simulink model "ODE_Hand_Model_v08_IPC_v03"  (Simulink 7.5)
settings: Solver=FixedStepDiscrete  StartTime=0.0  StopTime=inf  FixedStep=0.0315/(4*12)  RelTol=1e-3
values from neighbouring files (symbols this model uses):
  f_step = 0.7    [Set_Parameters.m]
  force_step = 20    [Set_Parameters.m]
  K_Conn = eye(4)*k_conn    [Set_Parameters.m]
  K_D = 30    [Set_Parameters.m]
  K_Or = eye(3)*k_Or    [Set_Parameters.m]
  K_Ot = eye(3)*k_Ot    [Set_Parameters.m]
  K_P = 350    [Set_Parameters.m]
  ksi = 0.9    [Set_Parameters.m]
  Kx = diag([diag(K_Ot)' diag(K_Or)' diag(K_Conn)'])    [Set_Parameters.m]
  l_des = [l1_des; l2_des; l3_des; l4_des]    [Set_Parameters.m]
  Mo = diag([sphere_mass*ones(1,3) (2/5)*sphere_mass*sphere_radius^2*ones(1,3)])    [Set_Parameters.m]
  qd_initial_touch = [0 0.3655   -0.5897   -0.5897     0       -0.3333   +0.5942   +0.5942         0       -0.298   --0.5226   --0.5226           0       -0.3333   +0.5942   +0.5942]    [Set_Parameters.m]
  R_O_Desired = R_O(x_i_v02(qd_initial_touch))    [Set_Parameters.m]
  t_f_start = 2.5    [Set_Parameters.m]
  torque_step = 60    [Set_Parameters.m]
  x_O_desired = (1/4)*sum(x_i_v02(qd_initial_touch))    [Set_Parameters.m]
undefined symbols (not defined in the file or in its folder): sigbuilder_block
libraries: dspmtrx3 x33, simulink x2, dspinverses x1
(part 1 of 6)
settings Model: Creator=konstantinos  LastModifiedBy=konstantinos
settings DataIOCC: SaveOutput=off  SaveTime=off
settings OptimizationCC: SimCompilerOptimization=On
settings SFSimCC: SFSimEnableDebug=off  SFSimOverflowDetection=off

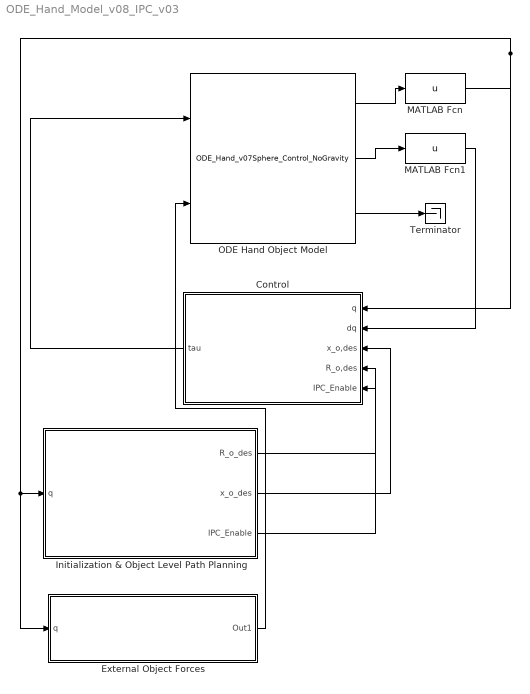
== system ODE_Hand_Model_v08_IPC_v03 ==
  Control : Subsystem
  External Object Forces : Subsystem
  Initialization & Object Level Path Planning : Subsystem
  MATLAB Fcn : MATLABFcn  MATLABFcn=u  Output1D=off
  MATLAB Fcn1 : MATLABFcn  MATLABFcn=u  Output1D=off
  ODE Hand Object Model : S-Function  FunctionName=ODE_Hand_v07Sphere_Control_NoGravity  EnableBusSupport=off
  Terminator : Terminator
  wires:
  Control/1(tau) -> ODE Hand Object Model/1
  Initialization & Object Level Path Planning/2(x_o_des) -> Control/3(x_o,des)
  Initialization & Object Level Path Planning/1(R_o_des) -> Control/4(R_o,des)
  Initialization & Object Level Path Planning/3(IPC_Enable) -> Control/5(IPC_Enable)
  ODE Hand Object Model/3 -> Terminator/1
  External Object Forces/1(Out1) -> ODE Hand Object Model/2
  ODE Hand Object Model/1 -> MATLAB Fcn/1
  MATLAB Fcn/1 -> Initialization & Object Level Path Planning/1(q), External Object Forces/1(q), Control/1(q)
  ODE Hand Object Model/2 -> MATLAB Fcn1/1
  MATLAB Fcn1/1 -> Control/2(dq)

== system ODE_Hand_Model_v08_IPC_v03/Control ==
  q : Inport  OutDataType=fixdt(1, 16)  OutScaling=2^0
  dq : Inport  Port=2  OutDataType=fixdt(1, 16)  OutScaling=2^0
  x_o,des : Inport  Port=3  OutDataType=fixdt(1, 16)  OutScaling=2^0
  R_o,des : Inport  Port=4  OutDataType=fixdt(1, 16)  OutScaling=2^0
  IPC_Enable : Inport  Port=5  OutDataType=fixdt(1, 16)  OutScaling=2^0
  IPC : Subsystem
  Initial_Posture : Subsystem
  Switch : Switch  OutDataType=fixdt(1, 16)  OutScaling=2^0
  tau : Outport  OutDataType=fixdt(1, 16)  OutScaling=2^0
  wires:
  Switch/1 -> tau/1
  x_o,des/1 -> IPC/3(x_o,des)
  R_o,des/1 -> IPC/4(R_o,des)
  IPC/1(tau) -> Switch/1
  IPC_Enable/1 -> Switch/2
  Initial_Posture/1(Out1) -> Switch/3
  q/1 -> IPC/1(q), Initial_Posture/1(q)
  dq/1 -> IPC/2(dq), Initial_Posture/2(dq)

== system ODE_Hand_Model_v08_IPC_v03/External Object Forces ==
  q : Inport  OutDataType=fixdt(1, 16)  OutScaling=2^0
  Apply Force : Subsystem
  Apply Torque : Subsystem
  Display : Display
  Force--Torque : simulink/Signal Routing/Manual Switch  SystemSampleTime=-1  sw=0  action=0  varsize=off
  Gain : Gain  Gain=0  ParameterDataType=fixdt(1, 16)  ParameterScaling=2^0  OutDataType=fixdt(1, 16)  OutScaling=2^0
  Mux1 : Mux
  Mux2 : Mux  Inputs=3
  Mux3 : Mux
  Object Gravity OFF1 : Constant  OutDataType=fixdt(1, 16)  OutScaling=2^0
  Object Gravity ON : Constant  Value=0  OutDataType=fixdt(1, 16)  OutScaling=2^0
  Object_Gravity OFF-ON : simulink/Signal Routing/Manual Switch  SystemSampleTime=-1  sw=1  action=0  varsize=off
  Zero_the Rest : Constant  Value=zeros(1,16-13)  OutDataType=fixdt(1, 16)  OutScaling=2^0
  Out1 : Outport  OutDataType=fixdt(1, 16)  OutScaling=2^0
  wires:
  Object Gravity OFF1/1 -> Object_Gravity OFF-ON/1
  Object Gravity ON/1 -> Object_Gravity OFF-ON/2
  Mux2/1 -> Out1/1, Display/1
  q/1 -> Apply Force/1(In1), Apply Torque/1(In1)
  Zero_the Rest/1 -> Mux2/3
  Object_Gravity OFF-ON/1 -> Mux2/2
  Mux1/1 -> Force--Torque/1
  Mux3/1 -> Force--Torque/2
  Apply Force/1(Out1) -> Mux1/1
  Apply Force/2(Out2) -> Mux1/2
  Apply Force/3(Out3) -> Mux1/3
  Apply Force/4(Out4) -> Mux1/4
  Apply Torque/1(Out1) -> Mux3/1
  Apply Torque/2(Out2) -> Mux3/2
  Apply Torque/3(Out3) -> Mux3/3
  Apply Torque/4(Out4) -> Mux3/4
  Force--Torque/1 -> Gain/1
  Gain/1 -> Mux2/1

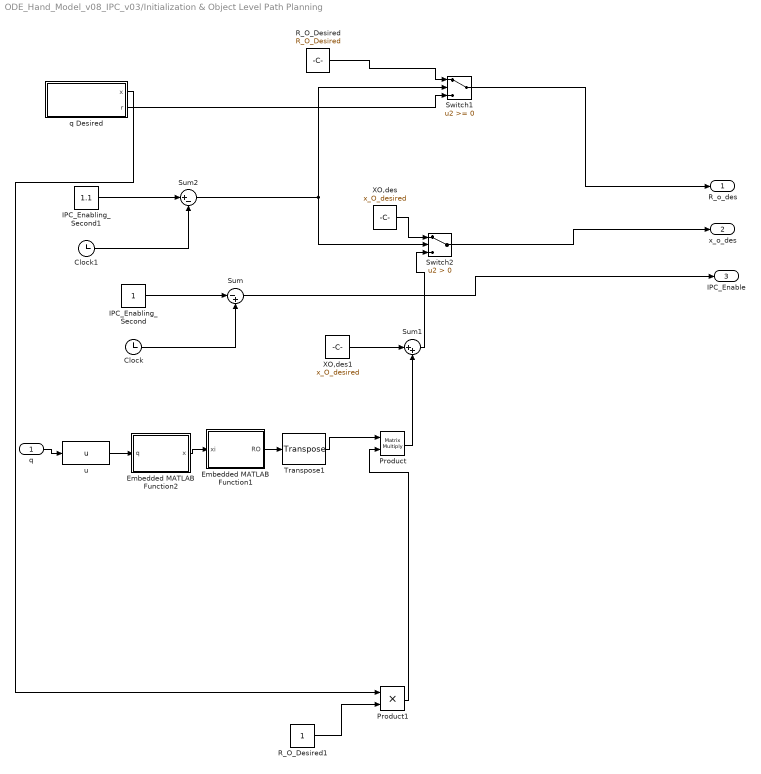
== system ODE_Hand_Model_v08_IPC_v03/Initialization & Object Level Path Planning ==
  q : Inport  OutDataType=fixdt(1, 16)  OutScaling=2^0
  Clock : Clock
      settings: Decimation=10
  Clock1 : Clock
      settings: Decimation=10
  Embedded MATLAB Function1 : Stateflow chart  TreatAsAtomicUnit=on
  Embedded MATLAB Function2 : Stateflow chart  TreatAsAtomicUnit=on
  IPC_Enabling_Second : Constant  OutDataType=fixdt(1, 16)  OutScaling=2^0
  IPC_Enabling_Second1 : Constant  Value=1.1  OutDataType=fixdt(1, 16)  OutScaling=2^0
  Product : Product  Multiplication=Matrix(*)  OutDataType=fixdt(1, 16)  OutScaling=2^0  RndMeth=Zero
  Product1 : Product  OutDataType=fixdt(1, 16)  OutScaling=2^0  RndMeth=Zero
  R_O_Desired : Constant  Value=R_O_Desired  OutDataType=fixdt(1, 16)  OutScaling=2^0
  R_O_Desired1 : Constant  OutDataType=fixdt(1, 16)  OutScaling=2^0
  Sum : Sum  Inputs=|-+  OutDataType=fixdt(1, 16)  OutScaling=2^0
  Sum1 : Sum  Inputs=|++  OutDataType=fixdt(1, 16)  OutScaling=2^0
  Sum2 : Sum  Inputs=|+-  OutDataType=fixdt(1, 16)  OutScaling=2^0
  Switch1 : Switch  OutDataType=fixdt(1, 16)  OutScaling=2^0
  Switch2 : Switch  Criteria=u2 > Threshold  OutDataType=fixdt(1, 16)  OutScaling=2^0
  Transpose1 : dspmtrx3/Transpose  SystemSampleTime=-1  Hermitian=off  overflowFlag=off
  XO,des : Constant  Value=x_O_desired  OutDataType=fixdt(1, 16)  OutScaling=2^0
  XO,des1 : Constant  Value=x_O_desired  OutDataType=fixdt(1, 16)  OutScaling=2^0
  q Desired : Subsystem
  u : MATLABFcn  MATLABFcn=u  Output1D=off
  R_o_des : Outport  OutDataType=fixdt(1, 16)  OutScaling=2^0
  x_o_des : Outport  Port=2  OutDataType=fixdt(1, 16)  OutScaling=2^0
  IPC_Enable : Outport  Port=3  OutDataType=fixdt(1, 16)  OutScaling=2^0
  wires:
  R_O_Desired/1 -> Switch1/1
  Switch2/1 -> x_o_des/1
  q/1 -> u/1
  Embedded MATLAB Function1/1(RO) -> Transpose1/1
  Sum1/1 -> Switch2/3
  XO,des/1 -> Switch2/1
  Product1/1 -> Product/2
  R_O_Desired1/1 -> Product1/2
  u/1 -> Embedded MATLAB Function2/1(q)
  Embedded MATLAB Function2/1(x) -> Embedded MATLAB Function1/1(xi)
  Clock/1 -> Sum/2
  IPC_Enabling_Second/1 -> Sum/1
  Sum/1 -> IPC_Enable/1
  XO,des1/1 -> Sum1/1
  Switch1/1 -> R_o_des/1
  Product/1 -> Sum1/2
  Clock1/1 -> Sum2/2
  IPC_Enabling_Second1/1 -> Sum2/1
  Sum2/1 -> Switch1/2, Switch2/2
  q Desired/1(x) -> Product1/1
  q Desired/2(r) -> Switch1/3
  Transpose1/1 -> Product/1

== system ODE_Hand_Model_v08_IPC_v03/Control/IPC ==
  q : Inport  OutDataType=fixdt(1, 16)  OutScaling=2^0
  dq : Inport  Port=2  OutDataType=fixdt(1, 16)  OutScaling=2^0
  x_o,des : Inport  Port=3  OutDataType=fixdt(1, 16)  OutScaling=2^0
  R_o,des : Inport  Port=4  OutDataType=fixdt(1, 16)  OutScaling=2^0
  Embedded MATLAB Function : Stateflow chart  TreatAsAtomicUnit=on
  Finger Redundancy Controller : Subsystem
  Gain : Gain  Gain=0  ParameterDataType=fixdt(1, 16)  ParameterScaling=2^0  OutDataType=fixdt(1, 16)  OutScaling=2^0
  J : Subsystem
  Object Level Damping(theta) : Subsystem
  "Object Level Stiffnes " : Subsystem
  Sum : Sum  Inputs=|---+  OutDataType=fixdt(1, 16)  OutScaling=2^0
  tau : Outport  OutDataType=fixdt(1, 16)  OutScaling=2^0
  wires:
  q/1 -> Object Level Damping(theta)/1(q), J/1(q), "Object Level Stiffnes "/1(q), Finger Redundancy Controller/1(q), Embedded MATLAB Function/1(theta_in)
  Sum/1 -> tau/1
  dq/1 -> Object Level Damping(theta)/3(dq), Finger Redundancy Controller/2(dq)
  "Object Level Stiffnes "/1(Out1) -> Sum/2
  Object Level Damping(theta)/1(Out1) -> Sum/3
  J/1(J_Ot) -> "Object Level Stiffnes "/2(J_Ot)
  J/2(J_Or) -> "Object Level Stiffnes "/3(J_Or)
  J/4(J_tot) -> Object Level Damping(theta)/2(J_tot)
  Finger Redundancy Controller/1(tau) -> Sum/1
  x_o,des/1 -> J/2(x_o,des), "Object Level Stiffnes "/5(x_o,des)
  J/3(JConn) -> "Object Level Stiffnes "/4(JConn)
  R_o,des/1 -> "Object Level Stiffnes "/6(R_o,des)
  Embedded MATLAB Function/1(gravity_dynamic_term) -> Gain/1
  Gain/1 -> Sum/4

== system ODE_Hand_Model_v08_IPC_v03/Control/Initial_Posture ==
  q : Inport  OutDataType=fixdt(1, 16)  OutScaling=2^0
  dq : Inport  Port=2  OutDataType=fixdt(1, 16)  OutScaling=2^0
  Gain : Gain  Gain=K_P  ParameterDataType=fixdt(1, 16)  ParameterScaling=2^0  OutDataType=fixdt(1, 16)  OutScaling=2^0
  Gain1 : Gain  Gain=K_D  ParameterDataType=fixdt(1, 16)  ParameterScaling=2^0  OutDataType=fixdt(1, 16)  OutScaling=2^0
  Ramp_Singals_qd : Subsystem
  Sum : Sum  Inputs=|--  OutDataType=fixdt(1, 16)  OutScaling=2^0
  Sum1 : Sum  Inputs=|-+  OutDataType=fixdt(1, 16)  OutScaling=2^0
  Out1 : Outport  OutDataType=fixdt(1, 16)  OutScaling=2^0
  wires:
  q/1 -> Sum1/2
  Sum/1 -> Out1/1
  Sum1/1 -> Gain/1
  dq/1 -> Gain1/1
  Gain1/1 -> Sum/1
  Gain/1 -> Sum/2
  Ramp_Singals_qd/1(Out1) -> Sum1/1

== system ODE_Hand_Model_v08_IPC_v03/External Object Forces/Apply Force ==
  In1 : Inport  OutDataType=fixdt(1, 16)  OutScaling=2^0
  Constant : Constant  Value=zeros(1,3)  VectorParams1D=off  OutDataType=fixdt(1, 16)  OutScaling=2^0
  Constant2 : Constant  Value=zeros(1,3)  VectorParams1D=off  OutDataType=fixdt(1, 16)  OutScaling=2^0
  Embedded MATLAB Function : Stateflow chart  TreatAsAtomicUnit=on
  Embedded MATLAB Function1 : Stateflow chart  TreatAsAtomicUnit=on
  Embedded MATLAB Function2 : Stateflow chart  TreatAsAtomicUnit=on
  F_x F_y F_z1 : Subsystem
  Transpose : dspmtrx3/Transpose  SystemSampleTime=-1  Hermitian=off  overflowFlag=off
  Out1 : Outport  OutDataType=fixdt(1, 16)  OutScaling=2^0
  Out2 : Outport  Port=2  OutDataType=fixdt(1, 16)  OutScaling=2^0
  Out3 : Outport  Port=3  OutDataType=fixdt(1, 16)  OutScaling=2^0
  Out4 : Outport  Port=4  OutDataType=fixdt(1, 16)  OutScaling=2^0
  wires:
  F_x F_y F_z1/1(Out1) -> Out2/1
  Embedded MATLAB Function/1(y) -> Out1/1
  Embedded MATLAB Function1/1(RO) -> Transpose/1
  Transpose/1 -> F_x F_y F_z1/1(xi)
  In1/1 -> Embedded MATLAB Function2/1(q)
  Constant/1 -> Out3/1
  Constant2/1 -> Out4/1
  Embedded MATLAB Function2/1(x) -> Embedded MATLAB Function1/1(xi), Embedded MATLAB Function/1(u)

== system ODE_Hand_Model_v08_IPC_v03/External Object Forces/Apply Torque ==
  In1 : Inport  OutDataType=fixdt(1, 16)  OutScaling=2^0
  Subsystem : Subsystem
  Subsystem2 : Subsystem
  Out1 : Outport  OutDataType=fixdt(1, 16)  OutScaling=2^0
  Out2 : Outport  Port=2  OutDataType=fixdt(1, 16)  OutScaling=2^0
  Out3 : Outport  Port=3  OutDataType=fixdt(1, 16)  OutScaling=2^0
  Out4 : Outport  Port=4  OutDataType=fixdt(1, 16)  OutScaling=2^0
  wires:
  Subsystem/1(Out1) -> Out1/1
  Subsystem/2(Out2) -> Out2/1
  Subsystem2/1(Out1) -> Out3/1
  Subsystem2/2(Out2) -> Out4/1
  In1/1 -> Subsystem/1(In1), Subsystem2/1(In1)

== system ODE_Hand_Model_v08_IPC_v03/Initialization & Object Level Path Planning/q Desired ==
  Discrete State-Space : DiscreteStateSpace  A=eye(3)  B=eye(3)  C=eye(3)  D=zeros(3)  X0=zeros(1,3)  SampleTime=0.0315/(4*12)
  Discrete State-Space1 : DiscreteStateSpace  A=eye(3)  B=eye(3)  C=eye(3)  D=zeros(3)  X0=zeros(1,3)  SampleTime=0.0315/(4*12)
  Embedded MATLAB Function : Stateflow chart  TreatAsAtomicUnit=on
  Level-2 M-file S-Function : M-S-Function  FunctionName=sfun_keyboard_input_v1_2
  MATLAB Fcn : MATLABFcn  MATLABFcn=R_O_Desired*rotx(u(1))*roty(u(2))*rotz(u(3))  Output1D=off
  MATLAB Fcn1 : MATLABFcn  MATLABFcn=u
  Product : Product  OutDataType=fixdt(1, 16)  OutScaling=2^0  RndMeth=Zero
  Transpose : dspmtrx3/Transpose  SystemSampleTime=-1  Hermitian=off  overflowFlag=off
  Transpose1 : dspmtrx3/Transpose  SystemSampleTime=-1  Hermitian=off  overflowFlag=off
  x : Outport  OutDataType=fixdt(1, 16)  OutScaling=2^0
  r : Outport  Port=2  OutDataType=fixdt(1, 16)  OutScaling=2^0
  wires:
  Level-2 M-file S-Function/2 -> Product/2
  Level-2 M-file S-Function/1 -> Product/1
  Product/1 -> Embedded MATLAB Function/1(key)
  Discrete State-Space1/1 -> MATLAB Fcn/1
  MATLAB Fcn/1 -> r/1
  MATLAB Fcn1/1 -> x/1
  Embedded MATLAB Function/1(x_f) -> Transpose/1
  Transpose/1 -> Discrete State-Space/1
  Embedded MATLAB Function/2(r_f) -> Transpose1/1
  Discrete State-Space/1 -> MATLAB Fcn1/1
  Transpose1/1 -> Discrete State-Space1/1

== system ODE_Hand_Model_v08_IPC_v03/Control/IPC/Finger Redundancy Controller ==
  q : Inport  OutDataType=fixdt(1, 16)  OutScaling=2^0
  dq : Inport  Port=2  OutDataType=fixdt(1, 16)  OutScaling=2^0
  Embedded MATLAB Function : Stateflow chart  TreatAsAtomicUnit=on
  tau : Outport  OutDataType=fixdt(1, 16)  OutScaling=2^0
  wires:
  dq/1 -> Embedded MATLAB Function/2(dq_in)
  q/1 -> Embedded MATLAB Function/1(q_in)
  Embedded MATLAB Function/1(tau_N) -> tau/1

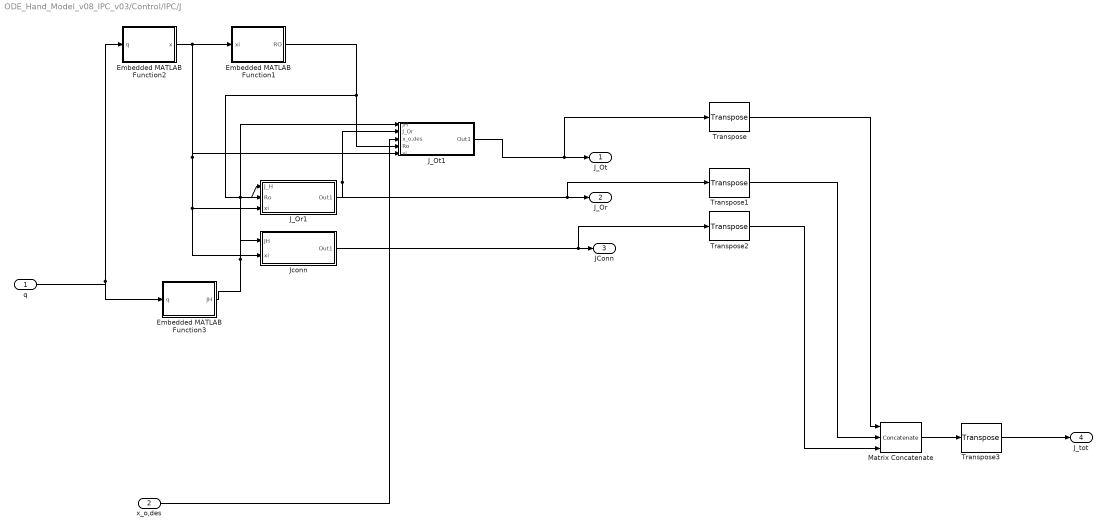
== system ODE_Hand_Model_v08_IPC_v03/Control/IPC/J ==
  q : Inport  OutDataType=fixdt(1, 16)  OutScaling=2^0
  x_o,des : Inport  Port=2  OutDataType=fixdt(1, 16)  OutScaling=2^0
  Embedded MATLAB Function1 : Stateflow chart  TreatAsAtomicUnit=on
  Embedded MATLAB Function2 : Stateflow chart  TreatAsAtomicUnit=on
  Embedded MATLAB Function3 : Stateflow chart  TreatAsAtomicUnit=on
  J_Or1 : Subsystem
  J_Ot1 : Subsystem
  Jconn : Subsystem
  Matrix Concatenate : Concatenate  NumInputs=3  Mode=Multidimensional array  ConcatenateDimension=2
  Transpose{,1..3} (4 alike) : dspmtrx3/Transpose  SystemSampleTime=-1  Hermitian=off  overflowFlag=off
  J_Ot : Outport  OutDataType=fixdt(1, 16)  OutScaling=2^0
  J_Or : Outport  Port=2  OutDataType=fixdt(1, 16)  OutScaling=2^0
  JConn : Outport  Port=3  OutDataType=fixdt(1, 16)  OutScaling=2^0
  J_tot : Outport  Port=4  OutDataType=fixdt(1, 16)  OutScaling=2^0
  wires:
  Embedded MATLAB Function3/1(JH) -> Jconn/1(JH), J_Or1/1(J_H), J_Ot1/1(JH)
  J_Or1/1(Out1) -> J_Ot1/2(J_Or), J_Or/1, Transpose1/1
  q/1 -> Embedded MATLAB Function2/1(q), Embedded MATLAB Function3/1(q)
  J_Ot1/1(Out1) -> J_Ot/1, Transpose/1
  Jconn/1(Out1) -> JConn/1, Transpose2/1
  Transpose2/1 -> Matrix Concatenate/3
  Transpose1/1 -> Matrix Concatenate/2
  Transpose/1 -> Matrix Concatenate/1
  Matrix Concatenate/1 -> Transpose3/1
  Transpose3/1 -> J_tot/1
  x_o,des/1 -> J_Ot1/3(x_o,des)
  Embedded MATLAB Function1/1(RO) -> J_Ot1/4(Ro), J_Or1/2(Ro)
  Embedded MATLAB Function2/1(x) -> J_Ot1/5(xi), J_Or1/3(xi), Jconn/2(xi), Embedded MATLAB Function1/1(xi)

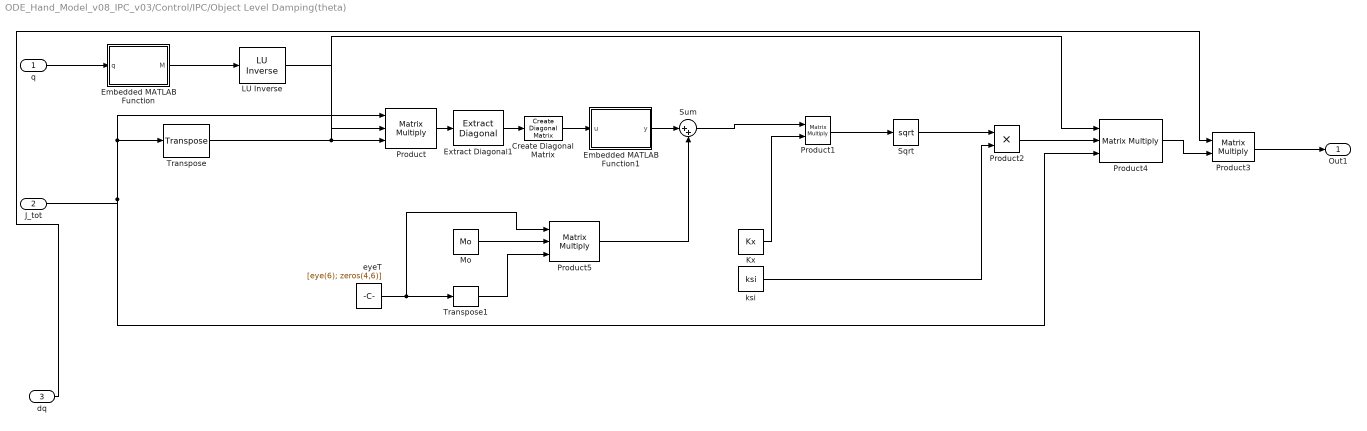
== system ODE_Hand_Model_v08_IPC_v03/Control/IPC/Object Level Damping(theta) ==
  q : Inport  OutDataType=fixdt(1, 16)  OutScaling=2^0
  J_tot : Inport  Port=2  OutDataType=fixdt(1, 16)  OutScaling=2^0
  dq : Inport  Port=3  OutDataType=fixdt(1, 16)  OutScaling=2^0
  " LU Inverse" : dspinverses/ LU Inverse  SystemSampleTime=-1
  Create Diagonal Matrix : dspmtrx3/Create Diagonal Matrix
  Embedded MATLAB Function : Stateflow chart  TreatAsAtomicUnit=on
  Embedded MATLAB Function1 : Stateflow chart  TreatAsAtomicUnit=on
  Extract Diagonal1 : dspmtrx3/Extract Diagonal
  Kx : Constant  Value=Kx  OutDataType=fixdt(1, 16)  OutScaling=2^0
  Mo : Constant  Value=Mo  OutDataType=fixdt(1, 16)  OutScaling=2^0
  Product : Product  Inputs=3  Multiplication=Matrix(*)  OutDataType=fixdt(1, 16)  OutScaling=2^0  RndMeth=Zero
  Product1 : Product  Multiplication=Matrix(*)  OutDataType=fixdt(1, 16)  OutScaling=2^0  RndMeth=Zero
  Product2 : Product  OutDataType=fixdt(1, 16)  OutScaling=2^0  RndMeth=Zero
  Product3 : Product  Multiplication=Matrix(*)  OutDataType=fixdt(1, 16)  OutScaling=2^0  RndMeth=Zero
  Product4 : Product  Inputs=3  Multiplication=Matrix(*)  OutDataType=fixdt(1, 16)  OutScaling=2^0  RndMeth=Zero
  Product5 : Product  Inputs=3  Multiplication=Matrix(*)  OutDataType=fixdt(1, 16)  OutScaling=2^0  RndMeth=Zero
  Sqrt : Sqrt  OutputSignalType=real  SaturateOnIntegerOverflow=on
  Sum : Sum  Inputs=|++  OutDataType=fixdt(1, 16)  OutScaling=2^0
  Transpose : dspmtrx3/Transpose  SystemSampleTime=-1  Hermitian=off  overflowFlag=off
  Transpose1 : dspmtrx3/Transpose  SystemSampleTime=-1  Hermitian=off  overflowFlag=off
  eyeT : Constant  Value=[eye(6); zeros(4,6)]  OutDataType=fixdt(1, 16)  OutScaling=2^0
  ksi : Constant  Value=ksi  OutDataType=fixdt(1, 16)  OutScaling=2^0
  Out1 : Outport  OutDataType=fixdt(1, 16)  OutScaling=2^0
  wires:
  q/1 -> Embedded MATLAB Function/1(q)
  J_tot/1 -> Transpose/1, Product/1, Product4/3
  Transpose/1 -> Product/3, Product4/1
  Embedded MATLAB Function/1(M) -> " LU Inverse"/1
  " LU Inverse"/1 -> Product/2
  Sqrt/1 -> Product2/1
  ksi/1 -> Product2/2
  Product2/1 -> Product4/2
  Product3/1 -> Out1/1
  Kx/1 -> Product1/2
  Product1/1 -> Sqrt/1
  eyeT/1 -> Transpose1/1, Product5/1
  Sum/1 -> Product1/1
  Mo/1 -> Product5/2
  Transpose1/1 -> Product5/3
  Product5/1 -> Sum/2
  Product/1 -> Extract Diagonal1/1
  Extract Diagonal1/1 -> Create Diagonal Matrix/1
  Create Diagonal Matrix/1 -> Embedded MATLAB Function1/1(u)
  Embedded MATLAB Function1/1(y) -> Sum/1
  Product4/1 -> Product3/2
  dq/1 -> Product3/1

== system ODE_Hand_Model_v08_IPC_v03/Control/IPC/Object Level Stiffnes  ==
  q : Inport  OutDataType=fixdt(1, 16)  OutScaling=2^0
  J_Ot : Inport  Port=2  OutDataType=fixdt(1, 16)  OutScaling=2^0
  J_Or : Inport  Port=3  OutDataType=fixdt(1, 16)  OutScaling=2^0
  JConn : Inport  Port=4  OutDataType=fixdt(1, 16)  OutScaling=2^0
  x_o,des : Inport  Port=5  OutDataType=fixdt(1, 16)  OutScaling=2^0
  R_o,des : Inport  Port=6  OutDataType=fixdt(1, 16)  OutScaling=2^0
  Embedded MATLAB Function1 : Stateflow chart  TreatAsAtomicUnit=on
  Embedded MATLAB Function2 : Stateflow chart  TreatAsAtomicUnit=on
  Sum : Sum  Inputs=|+++  OutDataType=fixdt(1, 16)  OutScaling=2^0
  VConn(theta) : Subsystem
  VO,r(theta) : Subsystem
  VO,t(theta) : Subsystem
  Out1 : Outport  OutDataType=fixdt(1, 16)  OutScaling=2^0
  wires:
  VO,r(theta)/1(Partial V_r) -> Sum/1
  Sum/1 -> Out1/1
  VO,t(theta)/1(Out1) -> Sum/2
  JConn/1 -> VConn(theta)/1(J_Conn)
  J_Ot/1 -> VO,t(theta)/1(JOt)
  J_Or/1 -> VO,r(theta)/1(JOr)
  x_o,des/1 -> VO,t(theta)/2(x_o,des)
  R_o,des/1 -> VO,r(theta)/2(R_o,des)
  VConn(theta)/1(Out1) -> Sum/3
  Embedded MATLAB Function2/1(x) -> Embedded MATLAB Function1/1(xi), VO,t(theta)/4(xi), VConn(theta)/2(xi)
  q/1 -> Embedded MATLAB Function2/1(q)
  Embedded MATLAB Function1/1(RO) -> VO,r(theta)/3(Ro), VO,t(theta)/3(Ro)

== system ODE_Hand_Model_v08_IPC_v03/Control/Initial_Posture/Ramp_Singals_qd ==
  Product : Product  OutDataType=fixdt(1, 16)  OutScaling=2^0  RndMeth=Zero
  Ramp : Subsystem  Tag=STV Subsys  LoadFcn=sigbuilder_block('load');  StartFcn=sigbuilder_block('start');  StopFcn=sigbuilder_block('stop');  ClipboardFcn=sigbuilder_block('clipboard');  mask(Sigbuilder block){}
      mask help: Create and generate interchangeable groups of signals whose waveforms are piecewise linear.
      mask init:
      | if ~strcmp(get_param(bdroot(gcbh),'SimulationStatus'),'stopped') tuvar = sigbuilder_block('maskInit'); end
      settings: CopyFcn=sigbuilder_block('copy');  DeleteFcn=sigbuilder_block('delete');  ModelCloseFcn=sigbuilder_block('modelClose');  PreSaveFcn=sigbuilder_block('preSave');  NameChangeFcn=sigbuilder_block('namechange');  OpenFcn=sigbuilder_block('open',[-1260 0 1260 730.5 ]);  CloseFcn=sigbuilder_block('close');
      mask Display: plot(0,0,100,100,[10,10,40,40,10],[80,20,20,80,80],[40,10],[50,50], [40,27,10],[65,72,56],[40,25,25,10],[28,28,43,43]);
  qd_initial_touch : Constant  Value=qd_initial_touch  OutDataType=fixdt(1, 16)  OutScaling=2^0
  Out1 : Outport  OutDataType=fixdt(1, 16)  OutScaling=2^0
  wires:
  Ramp/1(Signal 1) -> Product/1
  qd_initial_touch/1 -> Product/2
  Product/1 -> Out1/1

== system ODE_Hand_Model_v08_IPC_v03/External Object Forces/Apply Force/F_x F_y F_z1 ==
  xi : Inport  OutDataType=fixdt(1, 16)  OutScaling=2^0
  Constant : Constant  Value=0  OutDataType=fixdt(1, 16)  OutScaling=2^0
  Constant1 : Constant  Value=0  OutDataType=fixdt(1, 16)  OutScaling=2^0
  Fx Force Multiplier : Subsystem
  Mux : Mux  Inputs=3
  Product : Product  Multiplication=Matrix(*)  OutDataType=fixdt(1, 16)  OutScaling=2^0  RndMeth=Zero
  Out1 : Outport  OutDataType=fixdt(1, 16)  OutScaling=2^0
  wires:
  Mux/1 -> Product/2
  Product/1 -> Out1/1
  xi/1 -> Product/1
  Fx Force Multiplier/1(Out1) -> Mux/1
  Constant/1 -> Mux/2
  Constant1/1 -> Mux/3

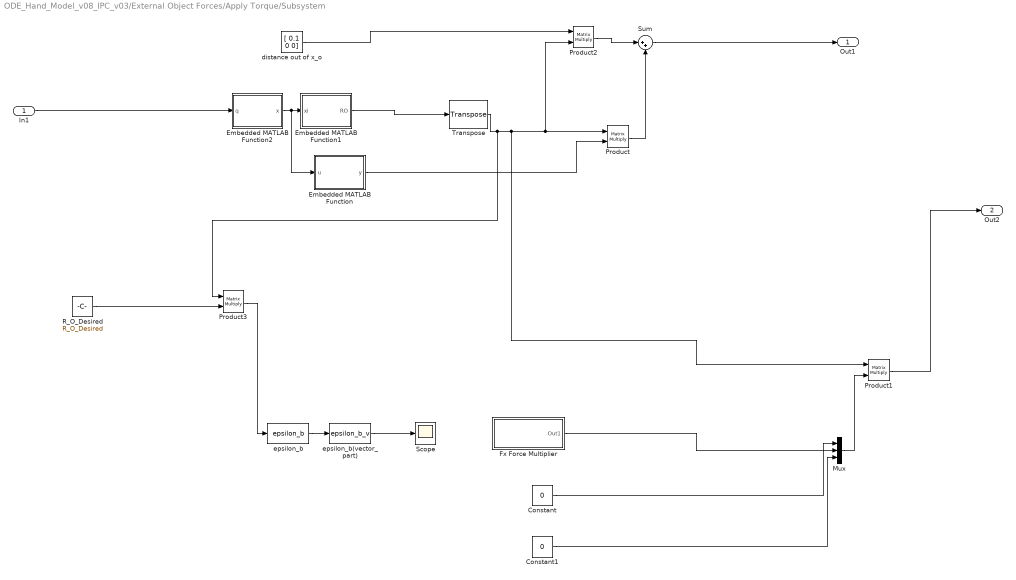
== system ODE_Hand_Model_v08_IPC_v03/External Object Forces/Apply Torque/Subsystem ==
  In1 : Inport  OutDataType=fixdt(1, 16)  OutScaling=2^0
  Constant : Constant  Value=0  OutDataType=fixdt(1, 16)  OutScaling=2^0
  Constant1 : Constant  Value=0  OutDataType=fixdt(1, 16)  OutScaling=2^0
  Embedded MATLAB Function : Stateflow chart  TreatAsAtomicUnit=on
  Embedded MATLAB Function1 : Stateflow chart  TreatAsAtomicUnit=on
  Embedded MATLAB Function2 : Stateflow chart  TreatAsAtomicUnit=on
  Fx Force Multiplier : Subsystem
  Mux : Mux  Inputs=3
  Product{,1..3} (4 alike) : Product  Multiplication=Matrix(*)  OutDataType=fixdt(1, 16)  OutScaling=2^0  RndMeth=Zero
  R_O_Desired : Constant  Value=R_O_Desired  OutDataType=fixdt(1, 16)  OutScaling=2^0
  Scope : Scope
      settings: YMin=-0.325  YMax=0.05  SaveName=e_b
  Sum : Sum  Inputs=|++  OutDataType=fixdt(1, 16)  OutScaling=2^0
  Transpose : dspmtrx3/Transpose  SystemSampleTime=-1  Hermitian=off  overflowFlag=off
  distance out of x_o : Constant  Value=[ 0.1 0 0]  VectorParams1D=off  OutDataType=fixdt(1, 16)  OutScaling=2^0
  epsilon_b : MATLABFcn  MATLABFcn=epsilon_b  Output1D=off
  epsilon_b(vector_part) : MATLABFcn  MATLABFcn=epsilon_b_v  Output1D=off
  Out1 : Outport  OutDataType=fixdt(1, 16)  OutScaling=2^0
  Out2 : Outport  Port=2  OutDataType=fixdt(1, 16)  OutScaling=2^0
  wires:
  Embedded MATLAB Function/1(y) -> Product/2
  Transpose/1 -> Product1/1, Product/1, Product2/2, Product3/1
  Product/1 -> Sum/2
  Mux/1 -> Product1/2
  distance out of x_o/1 -> Product2/1
  Product2/1 -> Sum/1
  Sum/1 -> Out1/1
  Product1/1 -> Out2/1
  Product3/1 -> epsilon_b/1
  epsilon_b/1 -> epsilon_b(vector_part)/1
  epsilon_b(vector_part)/1 -> Scope/1
  R_O_Desired/1 -> Product3/2
  Fx Force Multiplier/1(Out1) -> Mux/2
  Constant/1 -> Mux/1
  Constant1/1 -> Mux/3
  Embedded MATLAB Function2/1(x) -> Embedded MATLAB Function1/1(xi), Embedded MATLAB Function/1(u)
  Embedded MATLAB Function1/1(RO) -> Transpose/1
  In1/1 -> Embedded MATLAB Function2/1(q)

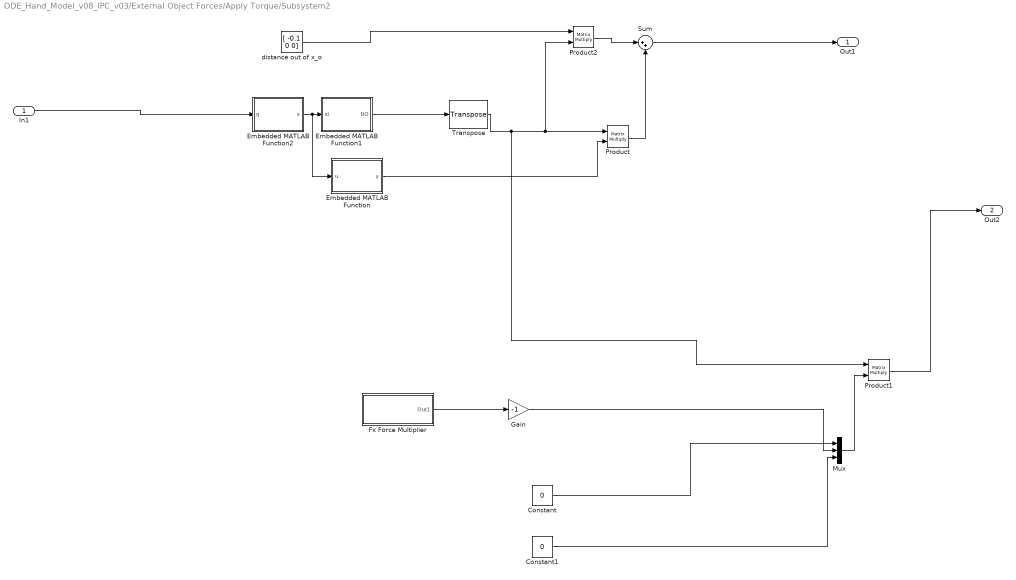
== system ODE_Hand_Model_v08_IPC_v03/External Object Forces/Apply Torque/Subsystem2 ==
  In1 : Inport  OutDataType=fixdt(1, 16)  OutScaling=2^0
  Constant : Constant  Value=0  OutDataType=fixdt(1, 16)  OutScaling=2^0
  Constant1 : Constant  Value=0  OutDataType=fixdt(1, 16)  OutScaling=2^0
  Embedded MATLAB Function : Stateflow chart  TreatAsAtomicUnit=on
  Embedded MATLAB Function1 : Stateflow chart  TreatAsAtomicUnit=on
  Embedded MATLAB Function2 : Stateflow chart  TreatAsAtomicUnit=on
  Fx Force Multiplier : Subsystem
  Gain : Gain  Gain=-1  ParameterDataType=fixdt(1, 16)  ParameterScaling=2^0  OutDataType=fixdt(1, 16)  OutScaling=2^0
  Mux : Mux  Inputs=3
  Product : Product  Multiplication=Matrix(*)  OutDataType=fixdt(1, 16)  OutScaling=2^0  RndMeth=Zero
  Product1 : Product  Multiplication=Matrix(*)  OutDataType=fixdt(1, 16)  OutScaling=2^0  RndMeth=Zero
  Product2 : Product  Multiplication=Matrix(*)  OutDataType=fixdt(1, 16)  OutScaling=2^0  RndMeth=Zero
  Sum : Sum  Inputs=|++  OutDataType=fixdt(1, 16)  OutScaling=2^0
  Transpose : dspmtrx3/Transpose  SystemSampleTime=-1  Hermitian=off  overflowFlag=off
  distance out of x_o : Constant  Value="[ -0.1 0   0]"  VectorParams1D=off  OutDataType=fixdt(1, 16)  OutScaling=2^0
  Out1 : Outport  OutDataType=fixdt(1, 16)  OutScaling=2^0
  Out2 : Outport  Port=2  OutDataType=fixdt(1, 16)  OutScaling=2^0
  wires:
  Transpose/1 -> Product1/1, Product/1, Product2/2
  Product/1 -> Sum/2
  Mux/1 -> Product1/2
  distance out of x_o/1 -> Product2/1
  Product2/1 -> Sum/1
  Sum/1 -> Out1/1
  Product1/1 -> Out2/1
  Fx Force Multiplier/1(Out1) -> Gain/1
  Constant/1 -> Mux/1
  Gain/1 -> Mux/2
  Constant1/1 -> Mux/3
  Embedded MATLAB Function2/1(x) -> Embedded MATLAB Function1/1(xi), Embedded MATLAB Function/1(u)
  Embedded MATLAB Function1/1(RO) -> Transpose/1
  In1/1 -> Embedded MATLAB Function2/1(q)
  Embedded MATLAB Function/1(y) -> Product/2

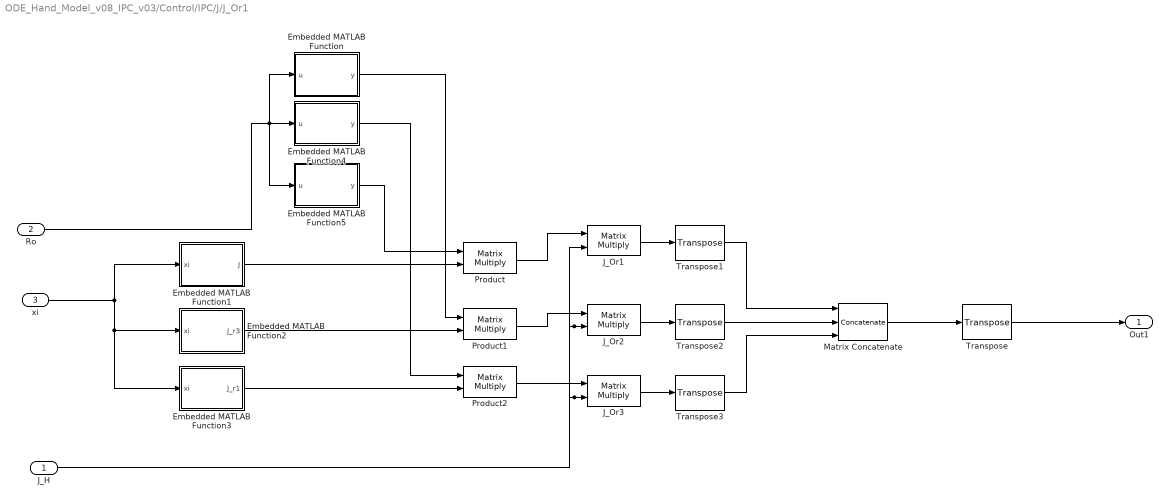
== system ODE_Hand_Model_v08_IPC_v03/Control/IPC/J/J_Or1 ==
  J_H : Inport  OutDataType=fixdt(1, 16)  OutScaling=2^0
  Ro : Inport  Port=2  OutDataType=fixdt(1, 16)  OutScaling=2^0
  xi : Inport  Port=3  OutDataType=fixdt(1, 16)  OutScaling=2^0
  Embedded MATLAB Function : Stateflow chart  TreatAsAtomicUnit=on
  Embedded MATLAB Function1 : Stateflow chart  TreatAsAtomicUnit=on
  Embedded MATLAB Function2 : Stateflow chart  TreatAsAtomicUnit=on
  Embedded MATLAB Function3 : Stateflow chart  TreatAsAtomicUnit=on
  Embedded MATLAB Function4 : Stateflow chart  TreatAsAtomicUnit=on
  Embedded MATLAB Function5 : Stateflow chart  TreatAsAtomicUnit=on
  J_Or1 : Product  Multiplication=Matrix(*)  OutDataType=fixdt(1, 16)  OutScaling=2^0  RndMeth=Zero
  J_Or2 : Product  Multiplication=Matrix(*)  OutDataType=fixdt(1, 16)  OutScaling=2^0  RndMeth=Zero
  J_Or3 : Product  Multiplication=Matrix(*)  OutDataType=fixdt(1, 16)  OutScaling=2^0  RndMeth=Zero
  Matrix Concatenate : Concatenate  NumInputs=3  Mode=Multidimensional array  ConcatenateDimension=2
  Product : Product  Multiplication=Matrix(*)  OutDataType=fixdt(1, 16)  OutScaling=2^0  RndMeth=Zero
  Product1 : Product  Multiplication=Matrix(*)  OutDataType=fixdt(1, 16)  OutScaling=2^0  RndMeth=Zero
  Product2 : Product  Multiplication=Matrix(*)  OutDataType=fixdt(1, 16)  OutScaling=2^0  RndMeth=Zero
  Transpose{,1..3} (4 alike) : dspmtrx3/Transpose  SystemSampleTime=-1  Hermitian=off  overflowFlag=off
  Out1 : Outport  OutDataType=fixdt(1, 16)  OutScaling=2^0
  wires:
  Product/1 -> J_Or1/1
  Product1/1 -> J_Or2/1
  Product2/1 -> J_Or3/1
  J_H/1 -> J_Or2/2, J_Or1/2, J_Or3/2
  Matrix Concatenate/1 -> Transpose/1
  Transpose/1 -> Out1/1
  J_Or1/1 -> Transpose1/1
  J_Or2/1 -> Transpose2/1
  J_Or3/1 -> Transpose3/1
  Transpose2/1 -> Matrix Concatenate/2
  Transpose1/1 -> Matrix Concatenate/1
  Transpose3/1 -> Matrix Concatenate/3
  Embedded MATLAB Function/1(y) -> Product1/1
  Embedded MATLAB Function4/1(y) -> Product2/1
  Embedded MATLAB Function5/1(y) -> Product/1
  Embedded MATLAB Function1/1(J) -> Product/2
  Embedded MATLAB Function2/1(J_r3) -> Product1/2
  Embedded MATLAB Function3/1(J_r1) -> Product2/2
  Ro/1 -> Embedded MATLAB Function/1(u), Embedded MATLAB Function4/1(u), Embedded MATLAB Function5/1(u)
  xi/1 -> Embedded MATLAB Function2/1(xi), Embedded MATLAB Function3/1(xi), Embedded MATLAB Function1/1(xi)

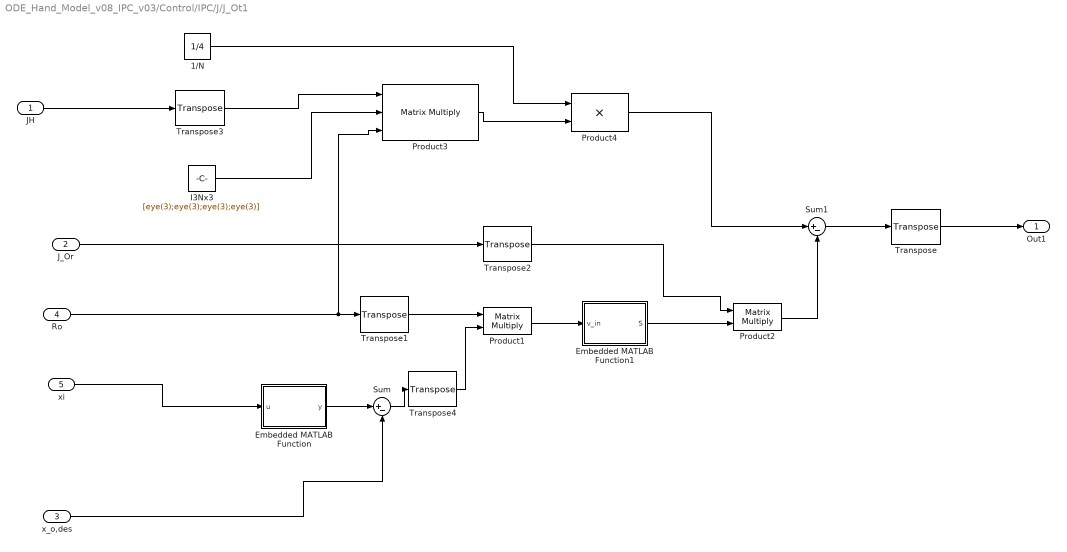
== system ODE_Hand_Model_v08_IPC_v03/Control/IPC/J/J_Ot1 ==
  JH : Inport  OutDataType=fixdt(1, 16)  OutScaling=2^0
  J_Or : Inport  Port=2  OutDataType=fixdt(1, 16)  OutScaling=2^0
  x_o,des : Inport  Port=3  OutDataType=fixdt(1, 16)  OutScaling=2^0
  Ro : Inport  Port=4  OutDataType=fixdt(1, 16)  OutScaling=2^0
  xi : Inport  Port=5  OutDataType=fixdt(1, 16)  OutScaling=2^0
  1/N : Constant  Value=1/4  OutDataType=fixdt(1, 16)  OutScaling=2^0
  Embedded MATLAB Function : Stateflow chart  TreatAsAtomicUnit=on
  Embedded MATLAB Function1 : Stateflow chart  TreatAsAtomicUnit=on
  I3Nx3 : Constant  Value=[eye(3);eye(3);eye(3);eye(3)]  OutDataType=fixdt(1, 16)  OutScaling=2^0
  Product1 : Product  Multiplication=Matrix(*)  OutDataType=fixdt(1, 16)  OutScaling=2^0  RndMeth=Zero
  Product2 : Product  Multiplication=Matrix(*)  OutDataType=fixdt(1, 16)  OutScaling=2^0  RndMeth=Zero
  Product3 : Product  Inputs=3  Multiplication=Matrix(*)  OutDataType=fixdt(1, 16)  OutScaling=2^0  RndMeth=Zero
  Product4 : Product  OutDataType=fixdt(1, 16)  OutScaling=2^0  RndMeth=Zero
  Sum : Sum  Inputs=|+-  OutDataType=fixdt(1, 16)  OutScaling=2^0
  Sum1 : Sum  Inputs=|+-  OutDataType=fixdt(1, 16)  OutScaling=2^0
  Transpose{,1..4} (5 alike) : dspmtrx3/Transpose  SystemSampleTime=-1  Hermitian=off  overflowFlag=off
  Out1 : Outport  OutDataType=fixdt(1, 16)  OutScaling=2^0
  wires:
  Ro/1 -> Transpose1/1, Product3/3
  Embedded MATLAB Function/1(y) -> Sum/1
  x_o,des/1 -> Sum/2
  Transpose1/1 -> Product1/1
  Product1/1 -> Embedded MATLAB Function1/1(v_in)
  Embedded MATLAB Function1/1(S) -> Product2/2
  J_Or/1 -> Transpose2/1
  Transpose2/1 -> Product2/1
  Product2/1 -> Sum1/2
  Sum1/1 -> Transpose/1
  Transpose/1 -> Out1/1
  JH/1 -> Transpose3/1
  Transpose3/1 -> Product3/1
  I3Nx3/1 -> Product3/2
  Product3/1 -> Product4/2
  Product4/1 -> Sum1/1
  1/N/1 -> Product4/1
  xi/1 -> Embedded MATLAB Function/1(u)
  Sum/1 -> Transpose4/1
  Transpose4/1 -> Product1/2

== system ODE_Hand_Model_v08_IPC_v03/Control/IPC/J/Jconn ==
  JH : Inport  OutDataType=fixdt(1, 16)  OutScaling=2^0
  xi : Inport  Port=2  OutDataType=fixdt(1, 16)  OutScaling=2^0
  Embedded MATLAB Function : Stateflow chart  TreatAsAtomicUnit=on
  Product2 : Product  Multiplication=Matrix(*)  OutDataType=fixdt(1, 16)  OutScaling=2^0  RndMeth=Zero
  Transpose : dspmtrx3/Transpose  SystemSampleTime=-1  Hermitian=off  overflowFlag=off
  Transpose1 : dspmtrx3/Transpose  SystemSampleTime=-1  Hermitian=off  overflowFlag=off
  Out1 : Outport  OutDataType=fixdt(1, 16)  OutScaling=2^0
  wires:
  Transpose/1 -> Product2/1
  JH/1 -> Transpose/1
  Product2/1 -> Transpose1/1
  Transpose1/1 -> Out1/1
  xi/1 -> Embedded MATLAB Function/1(xi)
  Embedded MATLAB Function/1(Jc) -> Product2/2

== system ODE_Hand_Model_v08_IPC_v03/Control/IPC/Object Level Stiffnes /VConn(theta) ==
  J_Conn : Inport  OutDataType=fixdt(1, 16)  OutScaling=2^0
  xi : Inport  Port=2  OutDataType=fixdt(1, 16)  OutScaling=2^0
  Embedded MATLAB Function : Stateflow chart  TreatAsAtomicUnit=on
  K_Conn : Constant  Value=K_Conn  OutDataType=fixdt(1, 16)  OutScaling=2^0
  Product : Product  Multiplication=Matrix(*)  OutDataType=fixdt(1, 16)  OutScaling=2^0  RndMeth=Zero
  Product1 : Product  Multiplication=Matrix(*)  OutDataType=fixdt(1, 16)  OutScaling=2^0  RndMeth=Zero
  Sum : Sum  Inputs=|+-  OutDataType=fixdt(1, 16)  OutScaling=2^0
  Transpose : dspmtrx3/Transpose  SystemSampleTime=-1  Hermitian=off  overflowFlag=off
  Transpose1 : dspmtrx3/Transpose  SystemSampleTime=-1  Hermitian=off  overflowFlag=off
  l_des : Constant  Value=l_des  OutDataType=fixdt(1, 16)  OutScaling=2^0
  Out1 : Outport  OutDataType=fixdt(1, 16)  OutScaling=2^0
  wires:
  Embedded MATLAB Function/1(Deltax) -> Sum/1
  l_des/1 -> Sum/2
  Sum/1 -> Product/2
  Product/1 -> Product1/2
  K_Conn/1 -> Product/1
  J_Conn/1 -> Transpose/1
  Transpose/1 -> Product1/1
  Product1/1 -> Transpose1/1
  Transpose1/1 -> Out1/1
  xi/1 -> Embedded MATLAB Function/1(xi)

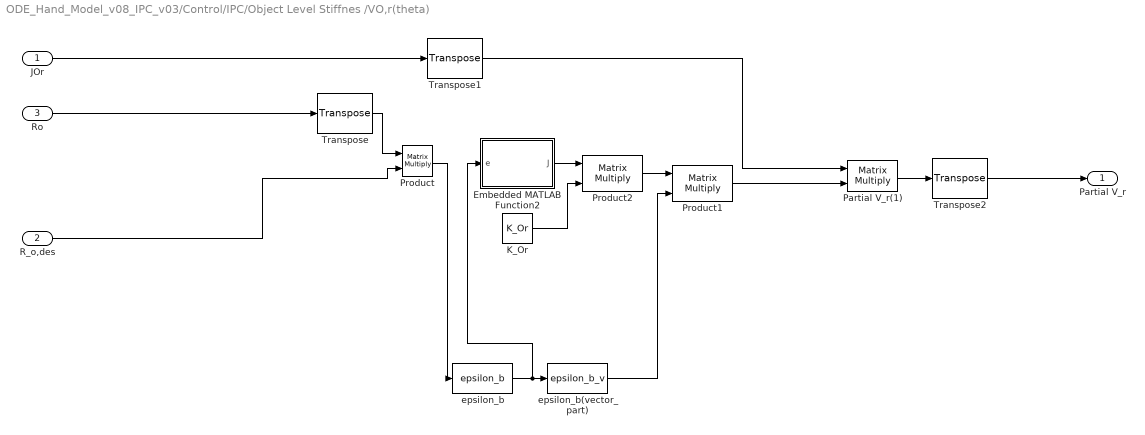
== system ODE_Hand_Model_v08_IPC_v03/Control/IPC/Object Level Stiffnes /VO,r(theta) ==
  JOr : Inport  OutDataType=fixdt(1, 16)  OutScaling=2^0
  R_o,des : Inport  Port=2  OutDataType=fixdt(1, 16)  OutScaling=2^0
  Ro : Inport  Port=3  OutDataType=fixdt(1, 16)  OutScaling=2^0
  Embedded MATLAB Function2 : Stateflow chart  TreatAsAtomicUnit=on
  K_Or : Constant  Value=K_Or  OutDataType=fixdt(1, 16)  OutScaling=2^0
  Partial V_r(1) : Product  Multiplication=Matrix(*)  OutDataType=fixdt(1, 16)  OutScaling=2^0  RndMeth=Zero
  Product : Product  Multiplication=Matrix(*)  OutDataType=fixdt(1, 16)  OutScaling=2^0  RndMeth=Zero
  Product1 : Product  Multiplication=Matrix(*)  OutDataType=fixdt(1, 16)  OutScaling=2^0  RndMeth=Zero
  Product2 : Product  Multiplication=Matrix(*)  OutDataType=fixdt(1, 16)  OutScaling=2^0  RndMeth=Zero
  Transpose : dspmtrx3/Transpose  SystemSampleTime=-1  Hermitian=off  overflowFlag=off
  Transpose1 : dspmtrx3/Transpose  SystemSampleTime=-1  Hermitian=off  overflowFlag=off
  Transpose2 : dspmtrx3/Transpose  SystemSampleTime=-1  Hermitian=off  overflowFlag=off
  epsilon_b : MATLABFcn  MATLABFcn=epsilon_b  Output1D=off
  epsilon_b(vector_part) : MATLABFcn  MATLABFcn=epsilon_b_v  Output1D=off
  Partial V_r : Outport  OutDataType=fixdt(1, 16)  OutScaling=2^0
  wires:
  Product1/1 -> Partial V_r(1)/2
  K_Or/1 -> Product2/2
  Product2/1 -> Product1/1
  Transpose1/1 -> Partial V_r(1)/1
  Ro/1 -> Transpose/1
  Transpose/1 -> Product/1
  JOr/1 -> Transpose1/1
  Partial V_r(1)/1 -> Transpose2/1
  Transpose2/1 -> Partial V_r/1
  Embedded MATLAB Function2/1(J) -> Product2/1
  R_o,des/1 -> Product/2
  epsilon_b/1 -> epsilon_b(vector_part)/1, Embedded MATLAB Function2/1(e)
  Product/1 -> epsilon_b/1
  epsilon_b(vector_part)/1 -> Product1/2

== system ODE_Hand_Model_v08_IPC_v03/Control/IPC/Object Level Stiffnes /VO,t(theta) ==
  JOt : Inport  OutDataType=fixdt(1, 16)  OutScaling=2^0
  x_o,des : Inport  Port=2  OutDataType=fixdt(1, 16)  OutScaling=2^0
  Ro : Inport  Port=3  OutDataType=fixdt(1, 16)  OutScaling=2^0
  xi : Inport  Port=4  OutDataType=fixdt(1, 16)  OutScaling=2^0
  Embedded MATLAB Function : Stateflow chart  TreatAsAtomicUnit=on
  K_Ot : Constant  Value=K_Ot  OutDataType=fixdt(1, 16)  OutScaling=2^0
  Product : Product  Multiplication=Matrix(*)  OutDataType=fixdt(1, 16)  OutScaling=2^0  RndMeth=Zero
  Product1 : Product  Multiplication=Matrix(*)  OutDataType=fixdt(1, 16)  OutScaling=2^0  RndMeth=Zero
  Product2 : Product  Multiplication=Matrix(*)  OutDataType=fixdt(1, 16)  OutScaling=2^0  RndMeth=Zero
  Sum : Sum  Inputs=|+-  OutDataType=fixdt(1, 16)  OutScaling=2^0
  Transpose : dspmtrx3/Transpose  SystemSampleTime=-1  Hermitian=off  overflowFlag=off
  Transpose1 : dspmtrx3/Transpose  SystemSampleTime=-1  Hermitian=off  overflowFlag=off
  Transpose2 : dspmtrx3/Transpose  SystemSampleTime=-1  Hermitian=off  overflowFlag=off
  Out1 : Outport  OutDataType=fixdt(1, 16)  OutScaling=2^0
  wires:
  JOt/1 -> Transpose/1
  Ro/1 -> Transpose1/1
  Embedded MATLAB Function/1(y) -> Sum/1
  Sum/1 -> Product1/2
  Product1/1 -> Product/2
  K_Ot/1 -> Product/1
  Product/1 -> Product2/2
  Transpose/1 -> Product2/1
  Product2/1 -> Transpose2/1
  Transpose2/1 -> Out1/1
  x_o,des/1 -> Sum/2
  Transpose1/1 -> Product1/1
  xi/1 -> Embedded MATLAB Function/1(u)

== system ODE_Hand_Model_v08_IPC_v03/Control/Initial_Posture/Ramp_Singals_qd/Ramp ==
  Demux : Demux  Tag=STV Demux  Outputs=1
  FromWs : FromWorkspace  Tag=STV FromWs  VariableName=tuvar  SampleTime=0  SigBuilderData=DataTag0  VnvData=DataTag1
      SigBuilderData=|
      | common.afterFinalStr = 'Extrapolate'
      | common.sampleTime = 0
      | dataSet.timeRange = [0 10]
      | dataSet.name = 'Group 1'
      | sbobj.Groups.Name = 'Group 1'
      | sbobj.Groups.Signals.Name = 'Signal 1'
      | sbobj.Groups.Signals.XData = [0 0.7 5 10]
      | sbobj.Groups.Signals.YData = [0 1 1 1]
  Signal 1 : Outport  Tag=STV Outport  OutDataType=fixdt(1, 16)  OutScaling=2^0
  wires:
  Demux/1 -> Signal 1/1
  FromWs/1 -> Demux/1

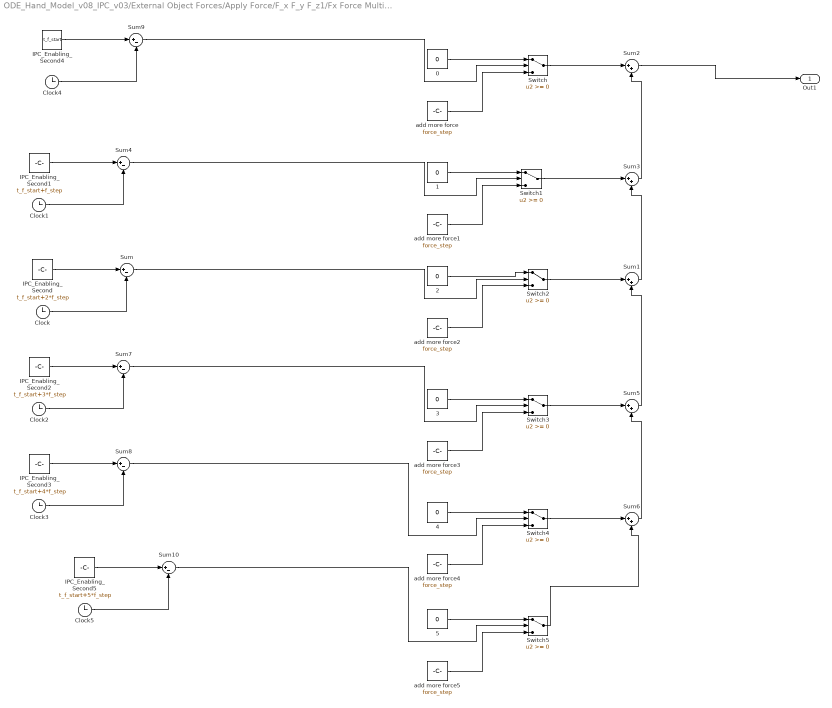
== system ODE_Hand_Model_v08_IPC_v03/External Object Forces/Apply Force/F_x F_y F_z1/Fx Force Multiplier ==
  {0..5} (6 alike) : Constant  Value=0  OutDataType=fixdt(1, 16)  OutScaling=2^0
  Clock{,1..5} (6 alike) : Clock
      settings: Decimation=10
  IPC_Enabling_Second : Constant  Value=t_f_start+2*f_step  OutDataType=fixdt(1, 16)  OutScaling=2^0
  IPC_Enabling_Second1 : Constant  Value=t_f_start+f_step  OutDataType=fixdt(1, 16)  OutScaling=2^0
  IPC_Enabling_Second2 : Constant  Value=t_f_start+3*f_step  OutDataType=fixdt(1, 16)  OutScaling=2^0
  IPC_Enabling_Second3 : Constant  Value=t_f_start+4*f_step  OutDataType=fixdt(1, 16)  OutScaling=2^0
  IPC_Enabling_Second4 : Constant  Value=t_f_start  OutDataType=fixdt(1, 16)  OutScaling=2^0
  IPC_Enabling_Second5 : Constant  Value=t_f_start+5*f_step  OutDataType=fixdt(1, 16)  OutScaling=2^0
  Sum{,4,7..10} (6 alike) : Sum  Inputs=|+-  OutDataType=fixdt(1, 16)  OutScaling=2^0
  Sum{1..3,5..6} (5 alike) : Sum  Inputs=|++  OutDataType=fixdt(1, 16)  OutScaling=2^0
  Switch{,1..5} (6 alike) : Switch  OutDataType=fixdt(1, 16)  OutScaling=2^0
  add more force{,1..5} (6 alike) : Constant  Value=force_step  OutDataType=fixdt(1, 16)  OutScaling=2^0
  Out1 : Outport  OutDataType=fixdt(1, 16)  OutScaling=2^0
  wires:
  0/1 -> Switch/1
  add more force/1 -> Switch/3
  Switch/1 -> Sum2/1
  1/1 -> Switch1/1
  add more force1/1 -> Switch1/3
  Switch1/1 -> Sum3/1
  2/1 -> Switch2/1
  add more force2/1 -> Switch2/3
  Switch2/1 -> Sum1/1
  add more force3/1 -> Switch3/3
  Switch3/1 -> Sum5/1
  4/1 -> Switch4/1
  add more force4/1 -> Switch4/3
  Switch4/1 -> Sum6/1
  5/1 -> Switch5/1
  add more force5/1 -> Switch5/3
  Switch5/1 -> Sum6/2
  Sum3/1 -> Sum2/2
  Sum1/1 -> Sum3/2
  Sum5/1 -> Sum1/2
  Sum6/1 -> Sum5/2
  Clock/1 -> Sum/2
  IPC_Enabling_Second/1 -> Sum/1
  Clock1/1 -> Sum4/2
  IPC_Enabling_Second1/1 -> Sum4/1
  Clock2/1 -> Sum7/2
  IPC_Enabling_Second2/1 -> Sum7/1
  Clock4/1 -> Sum9/2
  IPC_Enabling_Second4/1 -> Sum9/1
  Clock3/1 -> Sum8/2
  IPC_Enabling_Second3/1 -> Sum8/1
  Clock5/1 -> Sum10/2
  IPC_Enabling_Second5/1 -> Sum10/1
  Sum2/1 -> Out1/1
  Sum9/1 -> Switch/2
  Sum4/1 -> Switch1/2
  Sum/1 -> Switch2/2
  3/1 -> Switch3/1
  Sum7/1 -> Switch3/2
  Sum8/1 -> Switch4/2
  Sum10/1 -> Switch5/2

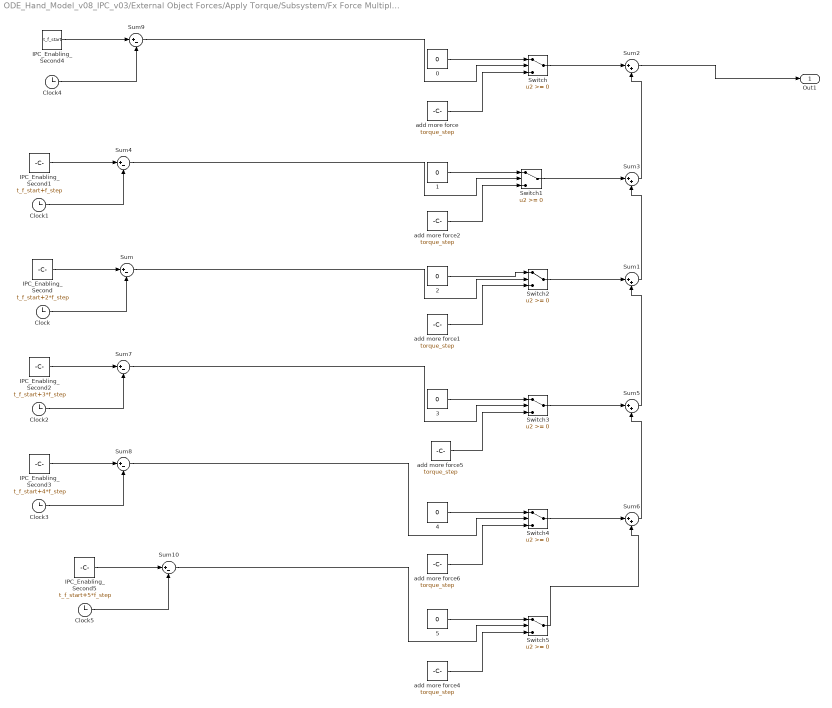
== system ODE_Hand_Model_v08_IPC_v03/External Object Forces/Apply Torque/Subsystem/Fx Force Multiplier ==
  {0..5} (6 alike) : Constant  Value=0  OutDataType=fixdt(1, 16)  OutScaling=2^0
  Clock{,1..5} (6 alike) : Clock
      settings: Decimation=10
  IPC_Enabling_Second : Constant  Value=t_f_start+2*f_step  OutDataType=fixdt(1, 16)  OutScaling=2^0
  IPC_Enabling_Second1 : Constant  Value=t_f_start+f_step  OutDataType=fixdt(1, 16)  OutScaling=2^0
  IPC_Enabling_Second2 : Constant  Value=t_f_start+3*f_step  OutDataType=fixdt(1, 16)  OutScaling=2^0
  IPC_Enabling_Second3 : Constant  Value=t_f_start+4*f_step  OutDataType=fixdt(1, 16)  OutScaling=2^0
  IPC_Enabling_Second4 : Constant  Value=t_f_start  OutDataType=fixdt(1, 16)  OutScaling=2^0
  IPC_Enabling_Second5 : Constant  Value=t_f_start+5*f_step  OutDataType=fixdt(1, 16)  OutScaling=2^0
  Sum{,4,7..10} (6 alike) : Sum  Inputs=|+-  OutDataType=fixdt(1, 16)  OutScaling=2^0
  Sum{1..3,5..6} (5 alike) : Sum  Inputs=|++  OutDataType=fixdt(1, 16)  OutScaling=2^0
  Switch{,1..5} (6 alike) : Switch  OutDataType=fixdt(1, 16)  OutScaling=2^0
  add more force{,1..2,4..6} (6 alike) : Constant  Value=torque_step  OutDataType=fixdt(1, 16)  OutScaling=2^0
  Out1 : Outport  OutDataType=fixdt(1, 16)  OutScaling=2^0
  wires:
  0/1 -> Switch/1
  add more force/1 -> Switch/3
  Switch/1 -> Sum2/1
  1/1 -> Switch1/1
  add more force2/1 -> Switch1/3
  Switch1/1 -> Sum3/1
  2/1 -> Switch2/1
  add more force1/1 -> Switch2/3
  Switch2/1 -> Sum1/1
  add more force5/1 -> Switch3/3
  Switch3/1 -> Sum5/1
  4/1 -> Switch4/1
  add more force6/1 -> Switch4/3
  Switch4/1 -> Sum6/1
  5/1 -> Switch5/1
  add more force4/1 -> Switch5/3
  Switch5/1 -> Sum6/2
  Sum3/1 -> Sum2/2
  Sum1/1 -> Sum3/2
  Sum5/1 -> Sum1/2
  Sum6/1 -> Sum5/2
  Clock/1 -> Sum/2
  IPC_Enabling_Second/1 -> Sum/1
  Clock1/1 -> Sum4/2
  IPC_Enabling_Second1/1 -> Sum4/1
  Clock2/1 -> Sum7/2
  IPC_Enabling_Second2/1 -> Sum7/1
  Clock4/1 -> Sum9/2
  IPC_Enabling_Second4/1 -> Sum9/1
  Clock3/1 -> Sum8/2
  IPC_Enabling_Second3/1 -> Sum8/1
  Clock5/1 -> Sum10/2
  IPC_Enabling_Second5/1 -> Sum10/1
  Sum2/1 -> Out1/1
  Sum9/1 -> Switch/2
  Sum4/1 -> Switch1/2
  Sum/1 -> Switch2/2
  3/1 -> Switch3/1
  Sum7/1 -> Switch3/2
  Sum8/1 -> Switch4/2
  Sum10/1 -> Switch5/2

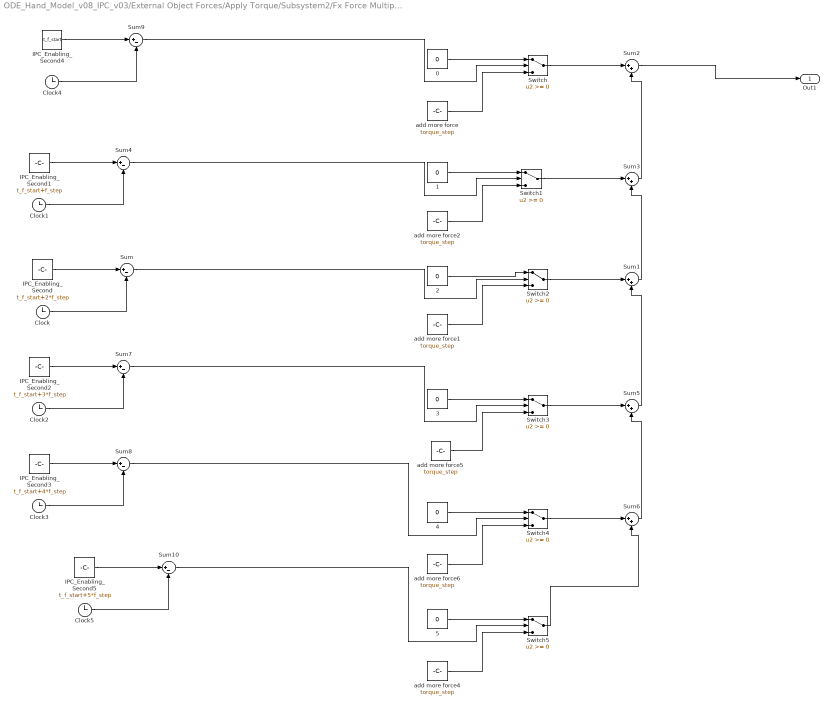
== system ODE_Hand_Model_v08_IPC_v03/External Object Forces/Apply Torque/Subsystem2/Fx Force Multiplier ==
  {0..5} (6 alike) : Constant  Value=0  OutDataType=fixdt(1, 16)  OutScaling=2^0
  Clock{,1..5} (6 alike) : Clock
      settings: Decimation=10
  IPC_Enabling_Second : Constant  Value=t_f_start+2*f_step  OutDataType=fixdt(1, 16)  OutScaling=2^0
  IPC_Enabling_Second1 : Constant  Value=t_f_start+f_step  OutDataType=fixdt(1, 16)  OutScaling=2^0
  IPC_Enabling_Second2 : Constant  Value=t_f_start+3*f_step  OutDataType=fixdt(1, 16)  OutScaling=2^0
  IPC_Enabling_Second3 : Constant  Value=t_f_start+4*f_step  OutDataType=fixdt(1, 16)  OutScaling=2^0
  IPC_Enabling_Second4 : Constant  Value=t_f_start  OutDataType=fixdt(1, 16)  OutScaling=2^0
  IPC_Enabling_Second5 : Constant  Value=t_f_start+5*f_step  OutDataType=fixdt(1, 16)  OutScaling=2^0
  Sum{,4,7..10} (6 alike) : Sum  Inputs=|+-  OutDataType=fixdt(1, 16)  OutScaling=2^0
  Sum{1..3,5..6} (5 alike) : Sum  Inputs=|++  OutDataType=fixdt(1, 16)  OutScaling=2^0
  Switch{,1..5} (6 alike) : Switch  OutDataType=fixdt(1, 16)  OutScaling=2^0
  add more force{,1..2,4..6} (6 alike) : Constant  Value=torque_step  OutDataType=fixdt(1, 16)  OutScaling=2^0
  Out1 : Outport  OutDataType=fixdt(1, 16)  OutScaling=2^0
  wires:
  0/1 -> Switch/1
  add more force/1 -> Switch/3
  Switch/1 -> Sum2/1
  1/1 -> Switch1/1
  add more force2/1 -> Switch1/3
  Switch1/1 -> Sum3/1
  2/1 -> Switch2/1
  add more force1/1 -> Switch2/3
  Switch2/1 -> Sum1/1
  add more force5/1 -> Switch3/3
  Switch3/1 -> Sum5/1
  4/1 -> Switch4/1
  add more force6/1 -> Switch4/3
  Switch4/1 -> Sum6/1
  5/1 -> Switch5/1
  add more force4/1 -> Switch5/3
  Switch5/1 -> Sum6/2
  Sum3/1 -> Sum2/2
  Sum1/1 -> Sum3/2
  Sum5/1 -> Sum1/2
  Sum6/1 -> Sum5/2
  Clock/1 -> Sum/2
  IPC_Enabling_Second/1 -> Sum/1
  Clock1/1 -> Sum4/2
  IPC_Enabling_Second1/1 -> Sum4/1
  Clock2/1 -> Sum7/2
  IPC_Enabling_Second2/1 -> Sum7/1
  Clock4/1 -> Sum9/2
  IPC_Enabling_Second4/1 -> Sum9/1
  Clock3/1 -> Sum8/2
  IPC_Enabling_Second3/1 -> Sum8/1
  Clock5/1 -> Sum10/2
  IPC_Enabling_Second5/1 -> Sum10/1
  Sum2/1 -> Out1/1
  Sum9/1 -> Switch/2
  Sum4/1 -> Switch1/2
  Sum/1 -> Switch2/2
  3/1 -> Switch3/1
  Sum7/1 -> Switch3/2
  Sum8/1 -> Switch4/2
  Sum10/1 -> Switch5/2

== matlab function Control/IPC/J/Embedded MATLAB Function1 ==
  data: xi input double size=[4 3]; RO output double
%#eml
function RO=R_O(xi)



x1 = xi(1,:);
x2 = xi(2,:);
x3 = xi(3,:);
x4 = xi(4,:);

% r1=( xi(1,:)-xi(3,:) )/norm( xi(1,:)-xi(3,:) ) + ...
%     ( xi(2,:)-xi(4,:) )/norm( xi(2,:)-xi(4,:) );

r1=( x1-x3 )/norm( x1-x3 ) + ...
    ( x2-x4 )/norm( x2-x4 );


r1_unit=r1/norm(r1);

% r3= cross( (x1-x3),( x2-x4 ))';

r3= skew( x1-x3 ) * ( x2-x4 )';
r3_unit=r3/norm(r3);

r2_unit = skew(r3_unit)*r1_unit';

l=[r1_unit' r2_unit r3_unit];
RO=l;

== matlab function Control/IPC/Object Level Stiffnes /Embedded MATLAB Function1 ==
  data: xi input double size=[4 3]; RO output double
%#eml
function RO=R_O(xi)



x1 = xi(1,:);
x2 = xi(2,:);
x3 = xi(3,:);
x4 = xi(4,:);

% r1=( xi(1,:)-xi(3,:) )/norm( xi(1,:)-xi(3,:) ) + ...
%     ( xi(2,:)-xi(4,:) )/norm( xi(2,:)-xi(4,:) );

r1=( x1-x3 )/norm( x1-x3 ) + ...
    ( x2-x4 )/norm( x2-x4 );


r1_unit=r1/norm(r1);

% r3= cross( (x1-x3),( x2-x4 ))';

r3= skew( x1-x3 ) * ( x2-x4 )';
r3_unit=r3/norm(r3);

r2_unit = skew(r3_unit)*r1_unit';

l=[r1_unit' r2_unit r3_unit];
RO=l;

== matlab function Control/IPC/J/Embedded MATLAB Function2 ==
  data: q input double; x output double
%#eml
function x=x_i_v02(q)

x_=zeros(4,3);

rot_base=[0.0000         0   -1.0000;
         0    1.0000         0;
    1.0000         0    0.0000];

L1 = 0.10;
L2 = 1.10;
L3 = 0.60;
L4 = 0.55;

fingers_positions = [-0.70,   0,  L1;...
                      0.60,  0.40,  L1;...
                      0.70,   0,  L1;...
                      0.60,  -0.40, L1];

c=1;
                  
for i=1:4:16,

q1 = q(i);
q2 = q(i+1);
q3 = q(i+2);
q4 = q(i+3);

x_(c,1)=cos(q1) .* (L2 .* cos(q2) + L3 .* cos(q2 + q3) + L4 .*  cos(q2 + q3 + q4));
x_(c,2)=(L2 .* cos(q2) + L3 .* cos(q2 + q3) + L4 .* cos(q2 + q3 + q4)) .* sin(q1);
x_(c,3)= L2 .* sin(q2) + L3 .* sin(q2 + q3) + L4 .* sin(q2 + q3 + q4);

x_(c,:)=rot_base*x_(c,:)'+fingers_positions(c,:)';
c=c+1;
end

x=x_;

== matlab function Control/IPC/Object Level Stiffnes /Embedded MATLAB Function2 ==
  data: q input double; x output double
%#eml
function x=x_i_v02(q)

x_=zeros(4,3);

rot_base=[0.0000         0   -1.0000;
         0    1.0000         0;
    1.0000         0    0.0000];

L1 = 0.10;
L2 = 1.10;
L3 = 0.60;
L4 = 0.55;

fingers_positions = [-0.70,   0,  L1;...
                      0.60,  0.40,  L1;...
                      0.70,   0,  L1;...
                      0.60,  -0.40, L1];

c=1;
                  
for i=1:4:16,

q1 = q(i);
q2 = q(i+1);
q3 = q(i+2);
q4 = q(i+3);

x_(c,1)=cos(q1) .* (L2 .* cos(q2) + L3 .* cos(q2 + q3) + L4 .*  cos(q2 + q3 + q4));
x_(c,2)=(L2 .* cos(q2) + L3 .* cos(q2 + q3) + L4 .* cos(q2 + q3 + q4)) .* sin(q1);
x_(c,3)= L2 .* sin(q2) + L3 .* sin(q2 + q3) + L4 .* sin(q2 + q3 + q4);

x_(c,:)=rot_base*x_(c,:)'+fingers_positions(c,:)';
c=c+1;
end

x=x_;

== matlab function Control/IPC/J/Embedded MATLAB Function3 ==
  data: q input double; JH output double
%#eml
function JH=J_H_v02(q)

J=zeros(12,16);

L2 = 1.10;
L3 = 0.60;
L4 = 0.55;

rot_base=[0.0000         0   -1.0000;
         0    1.0000         0;
    1.0000         0    0.0000];

c=1;
for i=1:4:16
q1 = q(i);
q2 = q(i+1);
q3 = q(i+2);
q4 = q(i+3);
    
    
J(c:c+2,i:i+3)=rot_base*[(-1) .* (L2 .* cos(q2) + L3 .* cos(q2 + q3) + L4 .* cos(q2 + q3 + ...
   q4)) .* sin(q1),(-1) .* cos(q1) .* (L2 .* sin(q2) + L3 .* sin(q2  ...
  + q3) + L4 .* sin(q2 + q3 + q4)),(-1) .* cos(q1) .* (L3 .* sin(q2  ...
  + q3) + L4 .* sin(q2 + q3 + q4)),(-1) .* L4 .* cos(q1) .* sin(q2 + ...
   q3 + q4);cos(q1) .* (L2 .* cos(q2) + L3 .* cos(q2 + q3) + L4 .*  ...
  cos(q2 + q3 + q4)),(-1) .* sin(q1) .* (L2 .* sin(q2) + L3 .* sin( ...
  q2 + q3) + L4 .* sin(q2 + q3 + q4)),(-1) .* sin(q1) .* (L3 .* sin( ...
  q2 + q3) + L4 .* sin(q2 + q3 + q4)),(-1) .* L4 .* sin(q1) .* sin( ...
  q2 + q3 + q4);0,cos(q1) .^ 2 .* (L2 .* cos(q2) + L3 .* cos(q2 +  ...
  q3) + L4 .* cos(q2 + q3 + q4)) + (L2 .* cos(q2) + L3 .* cos(q2 +  ...
  q3) + L4 .* cos(q2 + q3 + q4)) .* sin(q1) .^ 2,cos(q1) .* ((-1) .* ...
   L2 .* cos(q1) .* cos(q2) + cos(q1) .* (L2 .* cos(q2) + L3 .* cos( ...
  q2 + q3) + L4 .* cos(q2 + q3 + q4))) + sin(q1) .* ((-1) .* L2 .*  ...
  cos(q2) .* sin(q1) + (L2 .* cos(q2) + L3 .* cos(q2 + q3) + L4 .*  ...
  cos(q2 + q3 + q4)) .* sin(q1)),cos(q1) .* ((-1) .* cos(q1) .* (L2  ...
  .* cos(q2) + L3 .* cos(q2 + q3)) + cos(q1) .* (L2 .* cos(q2) + L3  ...
  .* cos(q2 + q3) + L4 .* cos(q2 + q3 + q4))) + sin(q1) .* ((-1) .*  ...
  (L2 .* cos(q2) + L3 .* cos(q2 + q3)) .* sin(q1) + (L2 .* cos(q2) + ...
   L3 .* cos(q2 + q3) + L4 .* cos(q2 + q3 + q4)) .* sin(q1))];

c=c+3;
end

JH=J;
